simulink library "ctrl_lib"  (R2017a)
settings: Solver=VariableStepAuto  StartTime=0.0  StopTime=10.0  RelTol=1e-3
undefined symbols (not defined in the file): DiscIntNeverNeededParam, low_lim, up_lim
libraries: ctrl_lib x3
settings Model: Creator=uids8840  LastModifiedBy=root

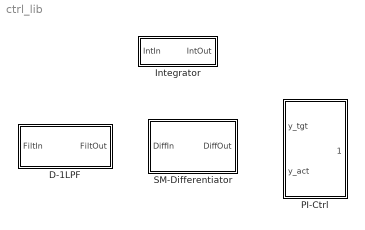
== system ctrl_lib ==
  D-1LPF : Subsystem  mask{k_filt=0.9615}
      mask prompts: k_filt "Filter Constant [tau / (tau + Ts)]:"
      mask DialogControl DescTextVar Prompt: Digital first order low pass filter.
  Integrator : Subsystem  SystemSampleTime=ts  mask{ts=1}
      mask prompts: ts "Execution Rate [s]:"
      mask DialogControl DescTextVar Prompt: ODE-1 Integrator.
  PI-Ctrl : Subsystem  SystemSampleTime=ts  mask{ts=1, PI_Kp=0, PI_Ki=0, PI_Max=inf, PI_Min=-inf}
      mask prompts: ts "Execution Rate [s]:"; PI_Kp "Proportional Gain:"; PI_Ki "Integral Gain:"; PI_Max "Upper limit"; PI_Min "Lower limit"
      mask DialogControl DescTextVar Prompt: Discrete PI Controller.
  SM-Differentiator : Subsystem  mask{sm_ki=1000, sm_kp=100, ts=1}
      mask prompts: sm_ki "Integral Gain:"; sm_kp "Proportional Gain:"; ts "Execution Rate [s]:"
      mask DialogControl DescTextVar Prompt: Second order sliding mode differentiator.

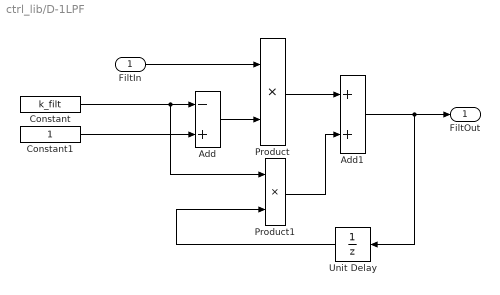
== system ctrl_lib/D-1LPF ==
  FiltIn : Inport
  Add : Sum  Inputs=-+
  Add1 : Sum
  Constant : Constant  Value=k_filt  OutDataTypeStr=Inherit: Inherit via back propagation
  Constant1 : Constant  OutDataTypeStr=Inherit: Inherit via back propagation
  Product : Product  OutDataTypeStr=Inherit: Same as first input
  Product1 : Product  OutDataTypeStr=Inherit: Same as first input
  Unit Delay : UnitDelay  SampleTime=-1
  FiltOut : Outport
  wires:
  Add1/1 -> FiltOut/1, Unit Delay/1
  FiltIn/1 -> Product/1
  Add/1 -> Product/2
  Product/1 -> Add1/1
  Unit Delay/1 -> Product1/2
  Constant/1 -> Product1/1, Add/1
  Constant1/1 -> Add/2
  Product1/1 -> Add1/2

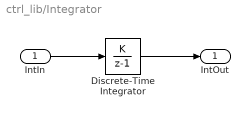
== system ctrl_lib/Integrator ==
  IntIn : Inport
  Discrete-Time Integrator : DiscreteIntegrator  IntegratorMethod=Accumulation: Forward Euler  gainval=ts  InitialConditionSetting=State (most efficient)  SampleTime=-1  UpperSaturationLimit=up_lim  LowerSaturationLimit=low_lim  ICPrevOutput=DiscIntNeverNeededParam  ICPrevScaledInput=DiscIntNeverNeededParam
  IntOut : Outport
  wires:
  IntIn/1 -> Discrete-Time Integrator/1
  Discrete-Time Integrator/1 -> IntOut/1

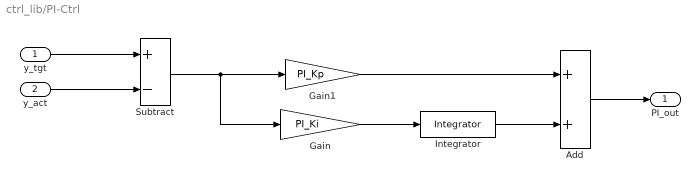
== system ctrl_lib/PI-Ctrl ==
  y_tgt : Inport
  y_act : Inport  Port=2
  Add : Sum  OutDataTypeStr=Inherit: Inherit via back propagation
  Gain : Gain  Gain=PI_Ki  ParamDataTypeStr=Inherit: Inherit from 'Gain'  OutDataTypeStr=Inherit: Inherit via back propagation
  Gain1 : Gain  Gain=PI_Kp  ParamDataTypeStr=Inherit: Inherit from 'Gain'  OutDataTypeStr=Inherit: Inherit via back propagation
  Integrator : ctrl_lib/Integrator  ts=ts
  Subtract : Sum  Inputs=+-
  PI_out : Outport
  wires:
  y_tgt/1 -> Subtract/1
  Gain1/1 -> Add/1
  y_act/1 -> Subtract/2
  Subtract/1 -> Gain/1, Gain1/1
  Gain/1 -> Integrator/1
  Integrator/1 -> Add/2
  Add/1 -> PI_out/1

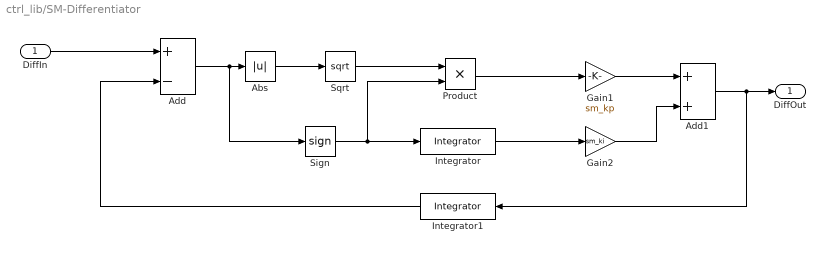
== system ctrl_lib/SM-Differentiator ==
  DiffIn : Inport
  Abs : Abs
  Add : Sum  Inputs=+-
  Add1 : Sum  OutDataTypeStr=Inherit: Inherit via back propagation
  Gain1 : Gain  Gain=sm_kp  ParamDataTypeStr=Inherit: Inherit from 'Gain'  OutDataTypeStr=Inherit: Inherit via back propagation
  Gain2 : Gain  Gain=sm_ki  ParamDataTypeStr=Inherit: Inherit from 'Gain'  OutDataTypeStr=Inherit: Inherit via back propagation
  Integrator : ctrl_lib/Integrator  ts=ts
  Integrator1 : ctrl_lib/Integrator  ts=ts
  Product : Product  OutDataTypeStr=Inherit: Same as first input
  Sign : Signum
  Sqrt : Sqrt  SaturateOnIntegerOverflow=on
  DiffOut : Outport
  wires:
  Gain2/1 -> Add1/2
  Integrator1/1 -> Add/2
  Sign/1 -> Integrator/1, Product/2
  Sqrt/1 -> Product/1
  Add1/1 -> Integrator1/1, DiffOut/1
  DiffIn/1 -> Add/1
  Abs/1 -> Sqrt/1
  Gain1/1 -> Add1/1
  Integrator/1 -> Gain2/1
  Product/1 -> Gain1/1
  Add/1 -> Sign/1, Abs/1
